simulink model "PV_ARRAY_MODEL"  (R2014a)
settings: Solver=ode45  StartTime=0.0  StopTime=4  RelTol=1e-3
libraries: elec_lib x31, fl_lib x5, nesl_utility x3, simulink x2
settings Model: Creator=yatin_000  LastModifiedBy=yatin_000

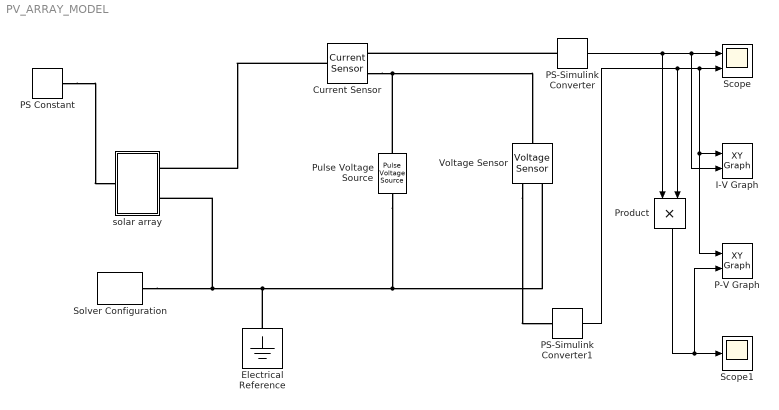
== system PV_ARRAY_MODEL ==
  Current Sensor : fl_lib/Electrical/Electrical Sensors/Current Sensor
  Electrical Reference : fl_lib/Electrical/Electrical Elements/Electrical Reference
  I-V Graph : simulink/Sinks/XY Graph  xmin=0  xmax=100  ymin=0  ymax=40  st=-1
  P-V Graph : simulink/Sinks/XY Graph  xmin=0  xmax=100  ymin=0  ymax=2000  st=-1
  PS Constant : fl_lib/Physical Signals/Sources/PS Constant  constant=1000
  PS-Simulink Converter : nesl_utility/PS-Simulink Converter  PhysicalDomain=network_engine_domain  SubClassName=ps_output  LeftPortType=input  RightPortType=output  PseudoPeriodic=off  Frequencies=[]  Unit=1  AffineConversion=off
  PS-Simulink Converter1 : nesl_utility/PS-Simulink Converter  PhysicalDomain=network_engine_domain  SubClassName=ps_output  LeftPortType=input  RightPortType=output  PseudoPeriodic=off  Frequencies=[]  Unit=1  AffineConversion=off
  Product : Product
  Pulse Voltage Source : elec_lib/Additional Components/SPICE-Compatible Components/Sources/Pulse Voltage Source  V1=0 V  V2=95 V  TD=0 s  TR=1 s  TF=1e-9 s  PW=Inf s  PER=Inf s
  Scope : Scope  NumInputPorts=2
      settings: YMin=-164.723~91.2  YMax=-149.035~100.8
  Scope1 : Scope
  Solver Configuration : nesl_utility/Solver Configuration  PhysicalDomain=network_engine_domain  SubClassName=solver  LeftPortType=input  RightPortType=generic  Accelerate=off  Tones=[]  Harmonics=[]  SimulateNoise=off  Profile=off  UseLocalSampling=off  EnableSwitchedLinearOptims=on  FrequencyDomain=off  UseCCode=off  RelTol=0.001  AbsTol=1e-06  MinStep=1e-09  ToWorkspace=off  DoDC=off  ResidualTolerance=1e-09  UseLocalSolver=on  LocalSolverChoice=NE_BACKWARD_EULER_ADVANCER  LocalSolverSampleTime=0.001  DoFixedCost=on  MaxNonlinIter=3  MaxModeIter=2  LinearAlgebra=Full  DelaysMemoryBudget=1024  AutomaticFiltering=off  FilteringTimeConstant=0.001
  Voltage Sensor : fl_lib/Electrical/Electrical Sensors/Voltage Sensor
  solar array : Subsystem
  wires:
  PS-Simulink Converter/1 -> Product/1, I-V Graph/2, Scope/1
  Product/1 -> P-V Graph/2, Scope1/1
  PS-Simulink Converter1/1 -> Product/2, I-V Graph/1, P-V Graph/1, Scope/2
  connections:
  Pulse Voltage Source/RConn1 -- Electrical Reference/LConn1 -- solar array/RConn2 -- Solver Configuration/RConn1 -- Voltage Sensor/RConn2
  Current Sensor/LConn1 -- solar array/RConn1
  Current Sensor/RConn2 -- Voltage Sensor/LConn1 -- Pulse Voltage Source/LConn1
  PS-Simulink Converter/LConn1 -- Current Sensor/RConn1
  Voltage Sensor/RConn1 -- PS-Simulink Converter1/LConn1
  PS Constant/RConn1 -- solar array/LConn1

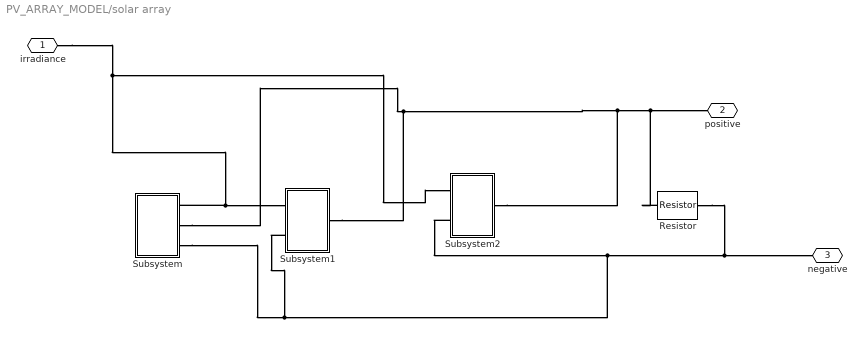
== system PV_ARRAY_MODEL/solar array ==
  Resistor : fl_lib/Electrical/Electrical Elements/Resistor  R=1000 Ohm  i_specify=off  i_priority=High  i=0 A  v_specify=off  v_priority=High  v=0 V
  Subsystem : Subsystem
  Subsystem1 : Subsystem
  Subsystem2 : Subsystem
  "irradiance " : PMIOPort  Port=1  Side=Left
  positive : PMIOPort  Port=2  Side=Right
  "negative " : PMIOPort  Port=3  Side=Right
  connections:
  Subsystem/RConn2 -- Subsystem1/RConn1 -- Subsystem2/RConn1 -- Resistor/LConn1 -- positive/RConn1
  Subsystem/RConn3 -- Subsystem1/LConn2 -- Subsystem2/LConn2 -- Resistor/RConn1 -- "negative "/RConn1
  Subsystem2/LConn1 -- "irradiance "/RConn1 -- Subsystem/RConn1 -- Subsystem1/LConn1

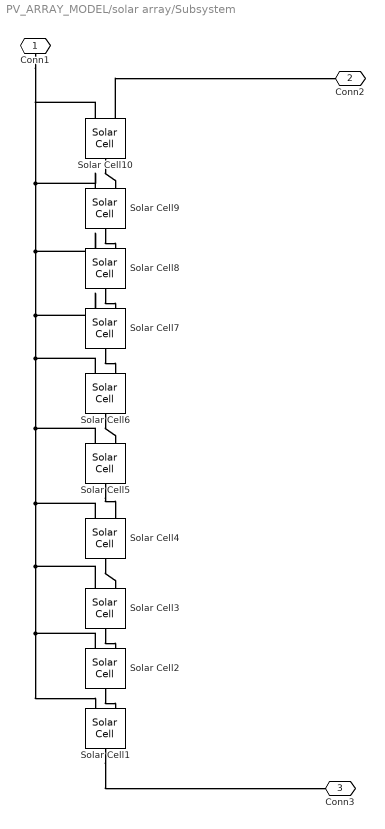
== system PV_ARRAY_MODEL/solar array/Subsystem ==
  Solar Cell{1..6,8..10} (9 alike) : elec_lib/Sources/Solar Cell  prm=1  Isc=7.34 A  Voc=0.8 V  Is=1e-6 A  Is2=0 A  Iph=7.34 A  Ir0=1000 W/m^2  ec=1.5  N2=2  Rs=0 Ohm  Rp=Inf Ohm  N_series=12  TIPH1=0 1/K  EG=1.11 eV  TXIS1=3  TXIS2=3  TRS1=0  TRP1=0  Tmeas=25 C  TFIXED=25 C  thermal_mass=100 J/K  initial_temperature=25 C
  Solar Cell7 : elec_lib/Sources/Solar Cell  prm=1  Isc=7.34 A  Voc=0.8 V  Is=1e-6 A  Is2=0 A  Iph=7.34 A  Ir0=1000 W/m^2  ec=1.5  N2=2  Rs=0 Ohm  Rp=Inf Ohm  N_series=1  TIPH1=0 1/K  EG=1.11 eV  TXIS1=3  TXIS2=3  TRS1=0  TRP1=0  Tmeas=25 C  TFIXED=25 C  thermal_mass=100 J/K  initial_temperature=25 C
  Conn1 : PMIOPort  Port=1  Side=Right
  Conn2 : PMIOPort  Port=2  Side=Right
  Conn3 : PMIOPort  Port=3  Side=Right
  connections:
  Solar Cell9/RConn1 -- Solar Cell8/LConn2
  Solar Cell2/RConn1 -- Solar Cell1/LConn2
  Solar Cell10/RConn1 -- Solar Cell9/LConn2
  Solar Cell4/RConn1 -- Solar Cell3/LConn2
  Solar Cell7/RConn1 -- Solar Cell6/LConn2
  Solar Cell5/RConn1 -- Solar Cell4/LConn2
  Solar Cell6/RConn1 -- Solar Cell5/LConn2
  Solar Cell3/RConn1 -- Solar Cell2/LConn2
  Solar Cell8/RConn1 -- Solar Cell7/LConn2
  Solar Cell6/LConn1 -- Conn1/RConn1 -- Solar Cell10/LConn1 -- Solar Cell9/LConn1 -- Solar Cell8/LConn1 -- Solar Cell7/LConn1 -- Solar Cell1/LConn1 -- Solar Cell2/LConn1 -- Solar Cell3/LConn1 -- Solar Cell4/LConn1 -- Solar Cell5/LConn1
  Solar Cell10/LConn2 -- Conn2/RConn1
  Solar Cell1/RConn1 -- Conn3/RConn1

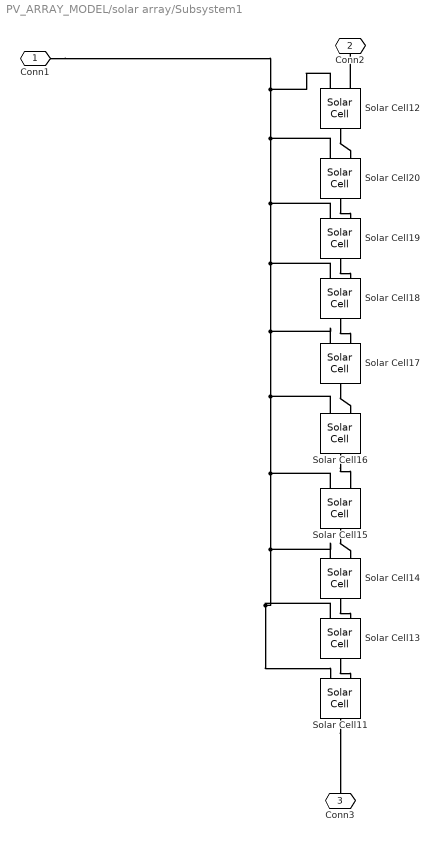
== system PV_ARRAY_MODEL/solar array/Subsystem1 ==
  Solar Cell{11..17,19..20} (9 alike) : elec_lib/Sources/Solar Cell  prm=1  Isc=7.34 A  Voc=0.8 V  Is=1e-6 A  Is2=0 A  Iph=7.34 A  Ir0=1000 W/m^2  ec=1.5  N2=2  Rs=0 Ohm  Rp=Inf Ohm  N_series=12  TIPH1=0 1/K  EG=1.11 eV  TXIS1=3  TXIS2=3  TRS1=0  TRP1=0  Tmeas=25 C  TFIXED=25 C  thermal_mass=100 J/K  initial_temperature=25 C
  Solar Cell18 : elec_lib/Sources/Solar Cell  prm=1  Isc=7.34 A  Voc=0.8 V  Is=1e-6 A  Is2=0 A  Iph=7.34 A  Ir0=1000 W/m^2  ec=1.5  N2=2  Rs=0 Ohm  Rp=Inf Ohm  N_series=1  TIPH1=0 1/K  EG=1.11 eV  TXIS1=3  TXIS2=3  TRS1=0  TRP1=0  Tmeas=25 C  TFIXED=25 C  thermal_mass=100 J/K  initial_temperature=25 C
  Conn1 : PMIOPort  Port=1  Side=Left
  Conn2 : PMIOPort  Port=2  Side=Right
  Conn3 : PMIOPort  Port=3  Side=Left
  connections:
  Solar Cell12/LConn2 -- Conn2/RConn1
  Solar Cell11/RConn1 -- Conn3/RConn1
  Solar Cell13/RConn1 -- Solar Cell11/LConn2
  Solar Cell19/RConn1 -- Solar Cell18/LConn2
  Solar Cell15/RConn1 -- Solar Cell14/LConn2
  Solar Cell12/LConn1 -- Conn1/RConn1 -- Solar Cell19/LConn1 -- Solar Cell18/LConn1 -- Solar Cell17/LConn1 -- Solar Cell16/LConn1 -- Solar Cell15/LConn1 -- Solar Cell14/LConn1 -- Solar Cell11/LConn1 -- Solar Cell13/LConn1 -- Solar Cell20/LConn1
  Solar Cell18/RConn1 -- Solar Cell17/LConn2
  Solar Cell12/RConn1 -- Solar Cell20/LConn2
  Solar Cell17/RConn1 -- Solar Cell16/LConn2
  Solar Cell14/RConn1 -- Solar Cell13/LConn2
  Solar Cell16/RConn1 -- Solar Cell15/LConn2
  Solar Cell20/RConn1 -- Solar Cell19/LConn2

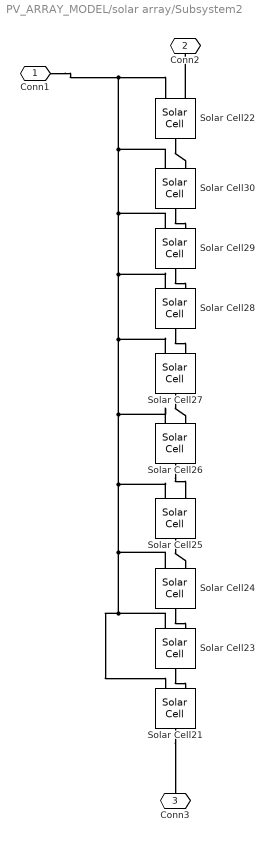
== system PV_ARRAY_MODEL/solar array/Subsystem2 ==
  Solar Cell{21..27,29..30} (9 alike) : elec_lib/Sources/Solar Cell  prm=1  Isc=7.34 A  Voc=0.8 V  Is=1e-6 A  Is2=0 A  Iph=7.34 A  Ir0=1000 W/m^2  ec=1.5  N2=2  Rs=0 Ohm  Rp=Inf Ohm  N_series=12  TIPH1=0 1/K  EG=1.11 eV  TXIS1=3  TXIS2=3  TRS1=0  TRP1=0  Tmeas=25 C  TFIXED=25 C  thermal_mass=100 J/K  initial_temperature=25 C
  Solar Cell28 : elec_lib/Sources/Solar Cell  prm=1  Isc=7.34 A  Voc=0.8 V  Is=1e-6 A  Is2=0 A  Iph=7.34 A  Ir0=1000 W/m^2  ec=1.5  N2=2  Rs=0 Ohm  Rp=Inf Ohm  N_series=1  TIPH1=0 1/K  EG=1.11 eV  TXIS1=3  TXIS2=3  TRS1=0  TRP1=0  Tmeas=25 C  TFIXED=25 C  thermal_mass=100 J/K  initial_temperature=25 C
  Conn1 : PMIOPort  Port=1  Side=Left
  Conn2 : PMIOPort  Port=2  Side=Right
  Conn3 : PMIOPort  Port=3  Side=Left
  connections:
  Solar Cell23/LConn1 -- Solar Cell21/LConn1 -- Solar Cell24/LConn1 -- Solar Cell25/LConn1 -- Solar Cell26/LConn1 -- Solar Cell27/LConn1 -- Solar Cell28/LConn1 -- Solar Cell30/LConn1 -- Conn1/RConn1 -- Solar Cell22/LConn1 -- Solar Cell29/LConn1
  Solar Cell21/RConn1 -- Conn3/RConn1
  Solar Cell22/LConn2 -- Conn2/RConn1
  Solar Cell22/RConn1 -- Solar Cell30/LConn2
  Solar Cell27/RConn1 -- Solar Cell26/LConn2
  Solar Cell25/RConn1 -- Solar Cell24/LConn2
  Solar Cell23/RConn1 -- Solar Cell21/LConn2
  Solar Cell29/RConn1 -- Solar Cell28/LConn2
  Solar Cell24/RConn1 -- Solar Cell23/LConn2
  Solar Cell26/RConn1 -- Solar Cell25/LConn2
  Solar Cell30/RConn1 -- Solar Cell29/LConn2
  Solar Cell28/RConn1 -- Solar Cell27/LConn2
